simulink model "buck"  (R2022b)
settings: Solver=VariableStepAuto  StartTime=0.0  StopTime=1  RelTol=1e-3
undefined symbols (not defined in the file): Ion, Lithium
libraries: spsDiodeLib x5, spsSeriesRLCBranchLib x3, spsCurrentMeasurementLib x3, spsACVoltageSourceLib x1, spsBatteryLib x1, spsIGBTDiodeLib x1, spsVoltageMeasurementLib x1, spspowerguiLib x1
settings Model: Creator=Dell  LastModifiedBy=ahmed
settings DebuggingCC: UnconnectedInputMsg=warning  UnconnectedOutputMsg=warning  UnconnectedLineMsg=warning
settings ModelReferenceCC: EnableRefExpFcnMdlSchedulingChecks=on
settings RTWCC: DLArmComputeVersion=19.05

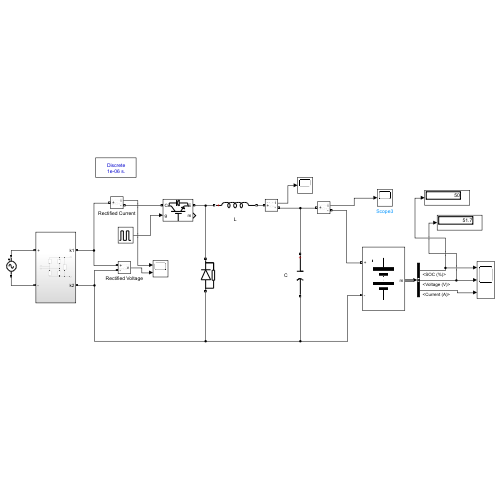
[thumbnail: Simulink's stored preview of the top-level diagram]
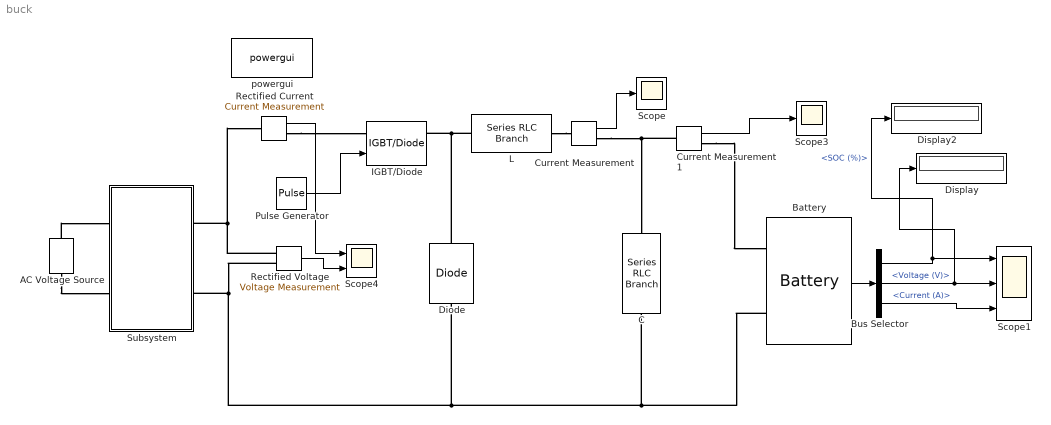
== system buck ==
  AC Voltage Source : spsACVoltageSourceLib/AC Voltage Source  Amplitude=72  Phase=0  Frequency=25000  SampleTime=0  Measurements=None  BusType=swing  Pref=10e3  Qref=0  Qmin=-inf  Qmax=+inf
  Battery : spsBatteryLib/Battery  BatType=Lithium-Ion  ShowTempParam=off  ThermalPreset=no  ShowAgeParam=off  NomV=48  NomQ=150  SOC=50  Batt_Tr=0.1  PresetModel=on  MaxQ=150  MinV=36  FullV=55.8714  Dis_rate=65.2174  R=0.0032  Normal_OP=135.6522  expZone="[51.8585      7.36957]"  current=[6.5 13 32.5]  Units=Time  Tci=20  NomT=20  T2=-30  MaxQ2=4.8  FullV2=7.1  Normal_OP2=5.655  expZone2="[6.58           1]"  Rca=0.6  ti=2000  Dp=0  Neq0=0  Tsim=1e6  Ta1=25  Qeol=5.4*0.9  Reol=0.013333*1.2  Char_age=[2.3478, 3]  Dis_age=[2.3478, 10]  N1=1500  N2=10500  N3=1000  N4=1400  Ta2=45  N5=950
  Bus Selector : BusSelector  OutputSignals=SOC (%),Voltage (V),Current (A)
  C : spsSeriesRLCBranchLib/Series RLC Branch  LConnTagsString=__new0  RConnTagsString=__new0  BranchType=C  Resistance=1  Inductance=1e-3  SetiL0=off  InitialCurrent=0  Capacitance=10e-6  Setx0=off  InitialVoltage=0  Measurements=None
  Current Measurement : spsCurrentMeasurementLib/Current Measurement  PhasorSimulation=off  OutputType=Complex  PSBequivalent=0
  Current Measurement1 : spsCurrentMeasurementLib/Current Measurement  PhasorSimulation=off  OutputType=Complex  PSBequivalent=0
  Diode : spsDiodeLib/Diode  Ron=0.001  Lon=0  Vf=0.8  IC=0  UseSnubber=0  Rs=500  Cs=250e-9  Measurements=off
  Display : Display
  Display2 : Display
  IGBT/Diode : spsIGBTDiodeLib/IGBT//Diode  Ron=1e-3  Rs=1e5  Cs=inf  Measurements=on
  L : spsSeriesRLCBranchLib/Series RLC Branch  LConnTagsString=__new0  RConnTagsString=__new0  BranchType=L  Resistance=1  Inductance=180e-6  SetiL0=off  InitialCurrent=0  Capacitance=1e-6  Setx0=off  InitialVoltage=0  Measurements=None
  Pulse Generator : DiscretePulseGenerator  PulseType=Time based  Period=1/20000  PulseWidth=30
  Rectified Current : spsCurrentMeasurementLib/Current Measurement  PhasorSimulation=off  OutputType=Complex  PSBequivalent=0
  Rectified Voltage : spsVoltageMeasurementLib/Voltage Measurement  PhasorSimulation=off  OutputType=Complex  PSBequivalent=0
  Scope : Scope
  Scope1 : Scope  NumInputPorts=3
  Scope3 : Scope
  Scope4 : Scope  NumInputPorts=2
  Subsystem : Subsystem
  powergui : spspowerguiLib/powergui  Priority=1  SimulationMode=Discrete  SampleTime=1e-6  frequency=60  Iterations=50  frequencyindice=0  Pbase=100e6  ErrMax=1e-4  UnitsV=kV  UnitsW=MW  buscounter=0  FunctionMessages=off  echomessages=off  EnableUseOfTLC=off  CurrentSourceSwitches=off  DisableSnubberDevices=off  DisableRonSwitches=off  DisableVfSwitches=off  DisplayEquations=off  AutomaticDiscreteSolvers=off  SolverType=Tustin/Backward Euler (TBE)  Interpol=off  ExternalGateDelay=off  methode=off  Ts=100  x0status=blocks  SPID=on  SwTol=0  HookPort=off  NonlinearTolerance=1e-4  nMaxIteration=100  ContinueOnMaxIteration=off  RestoreLinks=warning  ResistiveCurrentMeasurement=off  Frange=[0:2:500]  Ylog=off  Xlog=on  ShowGrid=off  save=off  variable=ZData  structure=0  ZoomFFT=off  StartTime=0.0  cycles=1  DisplayStyle=1  fundamental=60  FreqAxis=off  MaxFrequency=1000  frequencyindicesteady=1  RmsSteady=1  display=off
  wires:
  Current Measurement/1 -> Scope/1
  Current Measurement1/1 -> Scope3/1
  Battery/1 -> Bus Selector/1
  Bus Selector/1 -> Display2/1, Scope1/1  "<SOC (%)>"
  Bus Selector/2 -> Display/1, Scope1/2  "<Voltage (V)>"
  Bus Selector/3 -> Scope1/3  "<Current (A)>"
  Pulse Generator/1 -> IGBT/Diode/1
  Rectified Voltage/1 -> Scope4/2
  Rectified Current/1 -> Scope4/1
  connections:
  Diode/RConn1 -- L/LConn1 -- IGBT/Diode/RConn1
  Current Measurement/RConn1 -- Current Measurement1/LConn1 -- C/LConn1
  L/RConn1 -- Current Measurement/LConn1
  Current Measurement1/RConn1 -- Battery/LConn1
  C/RConn1 -- Battery/LConn2 -- Diode/LConn1 -- Rectified Voltage/LConn2 -- Subsystem/RConn2
  Rectified Current/RConn1 -- IGBT/Diode/LConn1
  Rectified Voltage/LConn1 -- Rectified Current/LConn1 -- Subsystem/RConn1
  AC Voltage Source/RConn1 -- Subsystem/LConn1
  AC Voltage Source/LConn1 -- Subsystem/LConn2

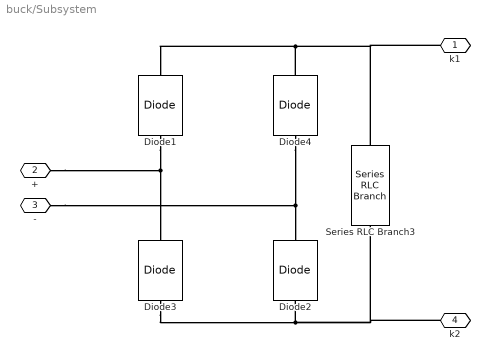
== system buck/Subsystem ==
  Diode{1..4} (4 alike) : spsDiodeLib/Diode  Ron=0.001  Lon=0  Vf=0.8  IC=0  UseSnubber=0  Rs=500  Cs=250e-9  Measurements=off
  Series RLC Branch3 : spsSeriesRLCBranchLib/Series RLC Branch  LConnTagsString=__new0  RConnTagsString=__new0  BranchType=C  Resistance=1  Inductance=1e-3  SetiL0=off  InitialCurrent=0  Capacitance=100e-6  Setx0=off  InitialVoltage=0  Measurements=None
  k1 : PMIOPort  Side=Right
  + : PMIOPort  Port=2  Side=Left
  - : PMIOPort  Port=3  Side=Left
  k2 : PMIOPort  Port=4  Side=Right
  connections:
  Diode1/LConn1 -- +/RConn1 -- Diode3/RConn1
  Diode4/RConn1 -- k1/RConn1 -- Series RLC Branch3/LConn1 -- Diode1/RConn1
  Diode3/LConn1 -- k2/RConn1 -- Series RLC Branch3/RConn1 -- Diode2/LConn1
  Diode4/LConn1 -- Diode2/RConn1 -- -/RConn1
